simulink model "bh_explore_car_eom"  (R2017b)
settings: Solver=ode45  StartTime=0.0  StopTime=30  FixedStep=0.001  RelTol=1e-5
undefined symbols (not defined in the file or in its folder): sigbuilder_block, veh
libraries: simulink_extras x15, bh_cv_car_drc_library x1
settings Model: Creator=bhorton  LastModifiedBy=bhorton
settings SolverCC: ZeroCrossControl=EnableAll  ZeroCrossAlgorithm=Adaptive
settings DebuggingCC: SignalInfNanChecking=warning
settings ModelReferenceCC: ModelReferenceMinAlgLoopOccurrences=on

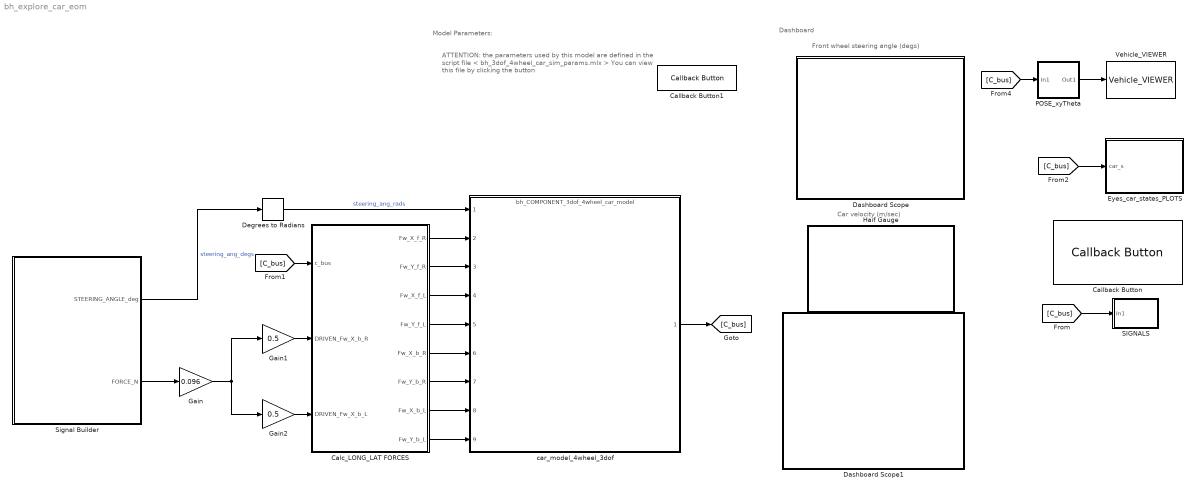
== system bh_explore_car_eom ==
  note: Car velocity (m/sec)
  note: ATTENTION:
      | the parameters used by this model are defined in the script file
      | < bh_3dof_4wheel_car_sim_params.mlx >
      |
      | You can view this file by clicking the button
  note: Model Parameters:
  note: Dashboard
  note: Front wheel steering angle (degs)
  Calc_LONG_LAT FORCES : Subsystem
  Callback Button : CallbackButton  WebBlockId=1673  PressFcn=""  ButtonText=OPEN State Plots  PressDelay=500  RepeatInterval=0
      settings: ClickFcn=|
      | open_system([bdroot,'/Eyes_car_states_PLOTS/car_states'])
      | open_system([bdroot,'/Eyes_car_states_PLOTS/Forces_BODY_frame'])
  Callback Button1 : CallbackButton  WebBlockId=1872  ButtonText=view parameter file  PressDelay=500  RepeatInterval=0
      settings: ClickFcn=edit bh_3dof_4wheel_car_sim_params.mlx
  Dashboard Scope : Subsystem  DialogController=hmiCreateDDGDialog  IsWebBlock=on  mask(MWDashboardBlock){webBlockId=37415055-6488-43ff-9aef-d1c13ce01a1d, webBlockType=sdiscope, ShowInitialText=on, HMISrcModelName=bh_explore_car_eom}
      mask prompts: webBlockId "WebBlock Id"; webBlockType "WebBlock Type"; HMISrcModelName "Source Model"
      mask help: SimulinkHMI:dialogs:HMIScopeDialogDesc
      mask Help: helpview([docroot '/mapfiles/simulink.map'], 'hmi_scope')
      mask Display:
      | if strcmp(get_param(bdroot(gcb),'BlockDiagramType'), 'library')
      |     image([(matlabroot) '/toolbox/simulink/hmi/icons/DashboardScope.png']);
      | end
  Dashboard Scope1 : Subsystem  DialogController=hmiCreateDDGDialog  IsWebBlock=on  mask(MWDashboardBlock){webBlockId=0f87227d-f9f9-4bc4-b6ae-007699aa5c2c, webBlockType=sdiscope, ShowInitialText=on, HMISrcModelName=bh_explore_car_eom}
      mask prompts: webBlockId "WebBlock Id"; webBlockType "WebBlock Type"; HMISrcModelName "Source Model"
      mask help: SimulinkHMI:dialogs:HMIScopeDialogDesc
      mask Help: helpview([docroot '/mapfiles/simulink.map'], 'hmi_scope')
      mask Display:
      | if strcmp(get_param(bdroot(gcb),'BlockDiagramType'), 'library')
      |     image([(matlabroot) '/toolbox/simulink/hmi/icons/DashboardScope.png']);
      | end
  Degrees to Radians : simulink_extras/Transformations/Degrees to Radians
  Eyes_car_states_PLOTS : Subsystem
  Gain : Gain  Gain=0.096
  Gain1 : Gain  Gain=0.5
  Gain2 : Gain  Gain=0.5
  Half Gauge : Subsystem  DialogController=hmiCreateDDGDialog  IsWebBlock=on  mask(MWDashboardBlock){webBlockId=0ce8c2a9-cad4-4196-9a6a-b4237871358c, webBlockType=semicirculargauge, ShowInLibBrowser=on, ShowInitialText=on, HMISrcModelName=bh_explore_car_eom}
      mask prompts: webBlockId "WebBlock Id"; webBlockType "WebBlock Type"; HMISrcModelName "Source Model"
      mask help: SimulinkHMI:dialogs:SemicircularGaugeDialogDesc
      mask Help: helpview([docroot '/mapfiles/simulink.map'], 'hmi_half_gauge')
      mask Display:
      | if strcmp(get_param(bdroot(gcb),'BlockDiagramType'), 'library')
      |     image([(matlabroot) '/toolbox/simulink/hmi/icons/SemicircularGauge.png']);
      | end
  POSE_xyTheta : Subsystem
  SIGNALS : Subsystem
  Signal Builder : Subsystem  Tag=STV Subsys  LoadFcn=sigbuilder_block('load');  StartFcn=sigbuilder_block('start');  StopFcn=sigbuilder_block('stop');  ClipboardFcn=sigbuilder_block('clipboard');  mask(Sigbuilder block){tuvar=[0:10]}
      mask help: Simulink:masks:SigbuilderBlock_MD
      mask init:
      | if ~strcmp(get_param(bdroot(gcbh),'SimulationStatus'),'stopped') tuvar = sigbuilder_block('maskInit'); end
      settings: CopyFcn=sigbuilder_block('copy');  DeleteFcn=sigbuilder_block('delete');  ModelCloseFcn=sigbuilder_block('modelClose');  PreSaveFcn=sigbuilder_block('preSave');  PauseFcn=sigbuilder_block('pause');  ContinueFcn=sigbuilder_block('continue');  NameChangeFcn=sigbuilder_block('namechange');  OpenFcn=sigbuilder_block('open',[437.6 199.2 550.4 400 ]);  CloseFcn=sigbuilder_block('close');
      mask Display: plot(0, 0, 100, 100,[2, 2, 32, 32, 2], [68, 8, 8, 68, 68],[32, 2], [38, 38], [32, 19, 2],[53, 60, 44], [32, 17, 17, 2],[16, 16, 31, 31]);txt = getActiveGroup(gcbh);text(2, 100, txt,'verticalAlignment', 'top');
  Vehicle_VIEWER : bh_cv_car_drc_library/CAR_things/Vehicle_VIEWER  wp_mat=[-1, -1; 2,2]  veh_ID_num=1  veh_init_xytheta=[0,0,0]  Ts=0.1
  car_model_4wheel_3dof : ModelReference  ModelNameDialog=bh_COMPONENT_3dof_4wheel_car_model.slx  SimulationMode=Normal  ModelReferenceVersion=1.187
  wires:
  [C_bus] -> Eyes_car_states_PLOTS/1(car_s)
  car_model_4wheel_3dof/1 -> [C_bus]
  [C_bus] -> POSE_xyTheta/1(In1)
  POSE_xyTheta/1(Out1) -> Vehicle_VIEWER/1
  [C_bus] -> SIGNALS/1(In1)
  Calc_LONG_LAT FORCES/8(Fw_Y_b_L) -> car_model_4wheel_3dof/9
  Calc_LONG_LAT FORCES/1(Fw_X_f_R) -> car_model_4wheel_3dof/2
  Calc_LONG_LAT FORCES/2(Fw_Y_f_R) -> car_model_4wheel_3dof/3
  Calc_LONG_LAT FORCES/3(Fw_X_f_L) -> car_model_4wheel_3dof/4
  Calc_LONG_LAT FORCES/4(Fw_Y_f_L) -> car_model_4wheel_3dof/5
  Calc_LONG_LAT FORCES/5(Fw_X_b_R) -> car_model_4wheel_3dof/6
  Calc_LONG_LAT FORCES/6(Fw_Y_b_R) -> car_model_4wheel_3dof/7
  Calc_LONG_LAT FORCES/7(Fw_X_b_L) -> car_model_4wheel_3dof/8
  [C_bus] -> Calc_LONG_LAT FORCES/1(c_bus)
  Degrees to Radians/1 -> car_model_4wheel_3dof/1  "steering_ang_rads"
  Gain/1 -> Gain1/1, Gain2/1
  Gain1/1 -> Calc_LONG_LAT FORCES/2(DRIVEN_Fw_X_b_R)
  Gain2/1 -> Calc_LONG_LAT FORCES/3(DRIVEN_Fw_X_b_L)
  Signal Builder/1(STEERING_ANGLE_deg) -> Degrees to Radians/1  "steering_ang_degs"
  Signal Builder/2(FORCE_N) -> Gain/1

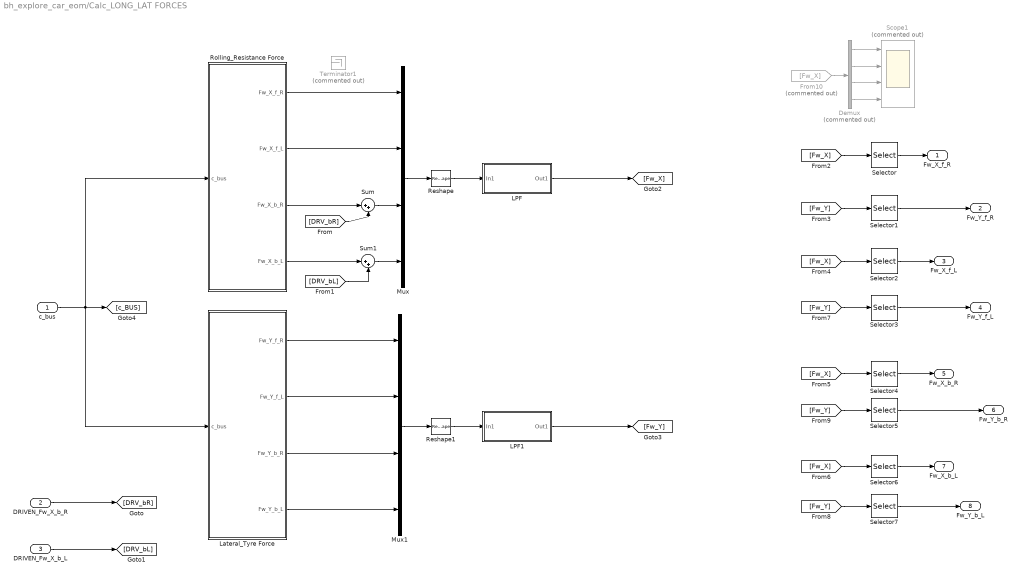
== system bh_explore_car_eom/Calc_LONG_LAT FORCES ==
  c_bus : Inport
  DRIVEN_Fw_X_b_R : Inport  Port=2
  DRIVEN_Fw_X_b_L : Inport  Port=3
  Demux : Demux  Commented=on
  From10 : From  Commented=on  GotoTag=Fw_X
  LPF : Subsystem
  LPF1 : Subsystem
  Lateral_Tyre Force : Subsystem
  Mux : Mux
  Mux1 : Mux
  Reshape : Reshape  OutputDimensionality=Column vector (2-D)
  Reshape1 : Reshape  OutputDimensionality=Column vector (2-D)
  Rolling_Resistance Force : Subsystem
  Scope1 : Scope  Commented=on  NumInputPorts=4
  Selector : Selector  InputPortWidth=4  IndexOptions=Index vector (dialog)  Indices=1  OutputSizes=1
  Selector1 : Selector  InputPortWidth=4  IndexOptions=Index vector (dialog)  Indices=1  OutputSizes=1
  Selector2 : Selector  InputPortWidth=4  IndexOptions=Index vector (dialog)  Indices=2  OutputSizes=1
  Selector3 : Selector  InputPortWidth=4  IndexOptions=Index vector (dialog)  Indices=2  OutputSizes=1
  Selector4 : Selector  InputPortWidth=4  IndexOptions=Index vector (dialog)  Indices=3  OutputSizes=1
  Selector5 : Selector  InputPortWidth=4  IndexOptions=Index vector (dialog)  Indices=3  OutputSizes=1
  Selector6 : Selector  InputPortWidth=4  IndexOptions=Index vector (dialog)  Indices=4  OutputSizes=1
  Selector7 : Selector  InputPortWidth=4  IndexOptions=Index vector (dialog)  Indices=4  OutputSizes=1
  Sum : Sum  Inputs=|++
  Sum1 : Sum  Inputs=|++
  Terminator1 : Terminator  Commented=on
  Fw_X_f_R : Outport
  Fw_Y_f_R : Outport  Port=2
  Fw_X_f_L : Outport  Port=3
  Fw_Y_f_L : Outport  Port=4
  Fw_X_b_R : Outport  Port=5
  Fw_Y_b_R : Outport  Port=6
  Fw_X_b_L : Outport  Port=7
  Fw_Y_b_L : Outport  Port=8
  wires:
  Selector/1 -> Fw_X_f_R/1
  Selector5/1 -> Fw_Y_b_R/1
  Selector7/1 -> Fw_Y_b_L/1
  Selector1/1 -> Fw_Y_f_R/1
  c_bus/1 -> [c_BUS], Rolling_Resistance Force/1(c_bus), Lateral_Tyre Force/1(c_bus)
  DRIVEN_Fw_X_b_R/1 -> [DRV_bR]
  DRIVEN_Fw_X_b_L/1 -> [DRV_bL]
  Rolling_Resistance Force/2(Fw_X_f_L) -> Mux/2
  Rolling_Resistance Force/1(Fw_X_f_R) -> Mux/1
  Lateral_Tyre Force/1(Fw_Y_f_R) -> Mux1/1
  Lateral_Tyre Force/2(Fw_Y_f_L) -> Mux1/2
  Lateral_Tyre Force/3(Fw_Y_b_R) -> Mux1/3
  Lateral_Tyre Force/4(Fw_Y_b_L) -> Mux1/4
  Mux1/1 -> Reshape1/1
  Mux/1 -> Reshape/1
  [Fw_Y] -> Selector1/1
  [Fw_X] -> Selector/1
  Selector6/1 -> Fw_X_b_L/1
  Selector4/1 -> Fw_X_b_R/1
  Selector3/1 -> Fw_Y_f_L/1
  Selector2/1 -> Fw_X_f_L/1
  [Fw_Y] -> Selector7/1
  [Fw_X] -> Selector6/1
  [Fw_Y] -> Selector5/1
  [Fw_X] -> Selector4/1
  [Fw_Y] -> Selector3/1
  [Fw_X] -> Selector2/1
  Reshape/1 -> LPF/1(In1)
  LPF/1(Out1) -> [Fw_X]
  LPF1/1(Out1) -> [Fw_Y]
  Demux/1 -> Scope1/1
  Demux/2 -> Scope1/2
  Demux/3 -> Scope1/3
  Demux/4 -> Scope1/4
  From10/1 -> Demux/1
  Rolling_Resistance Force/3(Fw_X_b_R) -> Sum/1
  [DRV_bR] -> Sum/2
  Sum1/1 -> Mux/4
  Rolling_Resistance Force/4(Fw_X_b_L) -> Sum1/1
  [DRV_bL] -> Sum1/2
  Sum/1 -> Mux/3
  Reshape1/1 -> LPF1/1(In1)

== system bh_explore_car_eom/Dashboard Scope ==

== system bh_explore_car_eom/Dashboard Scope1 ==

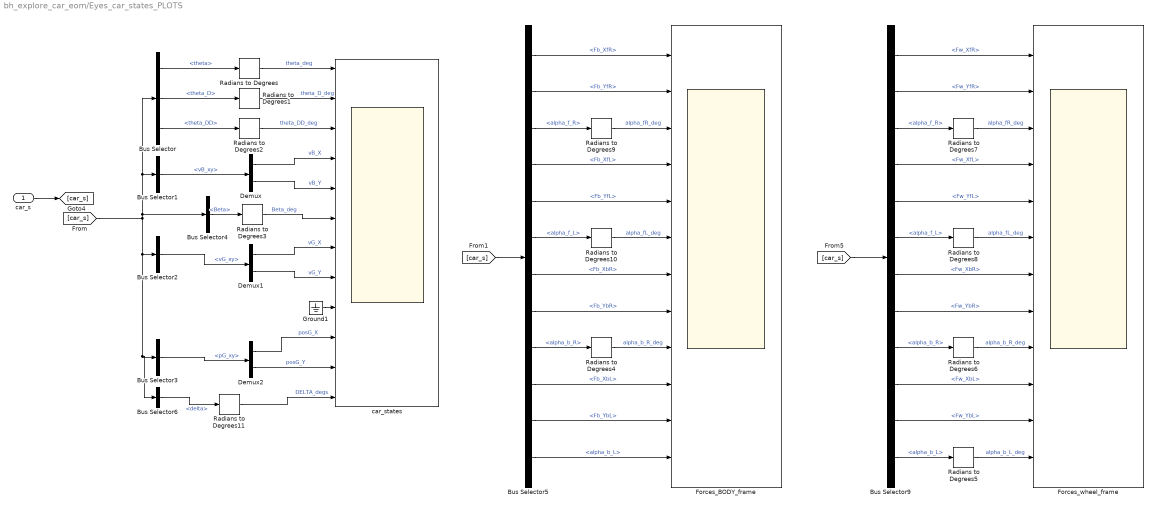
== system bh_explore_car_eom/Eyes_car_states_PLOTS ==
  car_s : Inport
  Bus Selector : BusSelector  OutputSignals=states_B.theta,states_B.theta_D,states_B.theta_DD
  Bus Selector1 : BusSelector  OutputSignals=states_B.vB_xy
  Bus Selector2 : BusSelector  OutputSignals=states_G.vG_xy
  Bus Selector3 : BusSelector  OutputSignals=states_G.pG_xy
  Bus Selector4 : BusSelector  OutputSignals=states_B.Beta
  Bus Selector5 : BusSelector  OutputSignals=Force_BODY_frame.Fb_XfR,Force_BODY_frame.Fb_YfR,alpha.alpha_f_R,Force_BODY_frame.Fb_XfL,Force_BODY_frame.Fb_YfL,alpha.alpha_f_L,Force_BODY_frame.Fb_XbR,Force_BODY_frame.Fb_YbR,alpha.alpha_b_R,Force_BODY_frame.Fb_XbL,Force_BODY_frame.Fb_YbL,alpha.alpha_b_L
  Bus Selector6 : BusSelector  OutputSignals=wheel.delta
  Bus Selector9 : BusSelector  OutputSignals=Force_wheel_frame.Fw_XfR,Force_wheel_frame.Fw_YfR,alpha.alpha_f_R,Force_wheel_frame.Fw_XfL,Force_wheel_frame.Fw_YfL,alpha.alpha_f_L,Force_wheel_frame.Fw_XbR,Force_wheel_frame.Fw_YbR,alpha.alpha_b_R,Force_wheel_frame.Fw_XbL,Force_wheel_frame.Fw_YbL,alpha.alpha_b_L
  Demux : Demux  Outputs=2
  Demux1 : Demux  Outputs=2
  Demux2 : Demux  Outputs=2
  Forces_BODY_frame : Scope  NumInputPorts=12
  Forces_wheel_frame : Scope  NumInputPorts=12
  Ground1 : Ground
  Radians to Degrees{,1..11} (12 alike) : simulink_extras/Transformations/Radians to Degrees
  car_states : Scope  NumInputPorts=12
  wires:
  car_s/1 -> [car_s]
  [car_s] -> Bus Selector4/1, Bus Selector/1, Bus Selector1/1, Bus Selector6/1, Bus Selector3/1, Bus Selector2/1
  Bus Selector/1 -> Radians to Degrees/1  "<theta>"
  Bus Selector/2 -> Radians to Degrees1/1  "<theta_D>"
  Bus Selector/3 -> Radians to Degrees2/1  "<theta_DD>"
  Radians to Degrees/1 -> car_states/1  "theta_deg"
  Radians to Degrees1/1 -> car_states/2  "theta_D_deg"
  Radians to Degrees2/1 -> car_states/3  "theta_DD_deg"
  Bus Selector1/1 -> Demux/1  "<vB_xy>"
  Demux/1 -> car_states/4  "vB_X"
  Demux/2 -> car_states/5  "vB_Y"
  Radians to Degrees3/1 -> car_states/6  "Beta_deg"
  Bus Selector2/1 -> Demux1/1  "<vG_xy>"
  Demux1/1 -> car_states/7  "vG_X"
  Demux1/2 -> car_states/8  "vG_Y"
  Ground1/1 -> car_states/9
  Demux2/1 -> car_states/10  "posG_X"
  Demux2/2 -> car_states/11  "posG_Y"
  Bus Selector3/1 -> Demux2/1  "<pG_xy>"
  Radians to Degrees11/1 -> car_states/12  "DELTA_degs"
  Bus Selector4/1 -> Radians to Degrees3/1  "<Beta>"
  [car_s] -> Bus Selector9/1
  Bus Selector9/1 -> Forces_wheel_frame/1  "<Fw_XfR>"
  Bus Selector9/2 -> Forces_wheel_frame/2  "<Fw_YfR>"
  Bus Selector9/3 -> Radians to Degrees7/1  "<alpha_f_R>"
  Bus Selector9/4 -> Forces_wheel_frame/4  "<Fw_XfL>"
  Bus Selector9/5 -> Forces_wheel_frame/5  "<Fw_YfL>"
  Bus Selector9/6 -> Radians to Degrees8/1  "<alpha_f_L>"
  Bus Selector9/7 -> Forces_wheel_frame/7  "<Fw_XbR>"
  Bus Selector9/8 -> Forces_wheel_frame/8  "<Fw_YbR>"
  Bus Selector9/9 -> Radians to Degrees6/1  "<alpha_b_R>"
  Bus Selector9/10 -> Forces_wheel_frame/10  "<Fw_XbL>"
  Bus Selector9/11 -> Forces_wheel_frame/11  "<Fw_YbL>"
  Bus Selector9/12 -> Radians to Degrees5/1  "<alpha_b_L>"
  Radians to Degrees7/1 -> Forces_wheel_frame/3  "alpha_fR_deg"
  Radians to Degrees8/1 -> Forces_wheel_frame/6  "alpha_fL_deg"
  Radians to Degrees6/1 -> Forces_wheel_frame/9  "alpha_b_R_deg"
  Radians to Degrees5/1 -> Forces_wheel_frame/12  "alpha_b_L_deg"
  Radians to Degrees10/1 -> Forces_BODY_frame/6  "alpha_fL_deg"
  Radians to Degrees4/1 -> Forces_BODY_frame/9  "alpha_b_R_deg"
  Radians to Degrees9/1 -> Forces_BODY_frame/3  "alpha_fR_deg"
  Bus Selector5/9 -> Radians to Degrees4/1  "<alpha_b_R>"
  Bus Selector5/7 -> Forces_BODY_frame/7  "<Fb_XbR>"
  Bus Selector5/10 -> Forces_BODY_frame/10  "<Fb_XbL>"
  Bus Selector5/11 -> Forces_BODY_frame/11  "<Fb_YbL>"
  Bus Selector5/6 -> Radians to Degrees10/1  "<alpha_f_L>"
  Bus Selector5/5 -> Forces_BODY_frame/5  "<Fb_YfL>"
  Bus Selector5/4 -> Forces_BODY_frame/4  "<Fb_XfL>"
  Bus Selector5/8 -> Forces_BODY_frame/8  "<Fb_YbR>"
  Bus Selector5/2 -> Forces_BODY_frame/2  "<Fb_YfR>"
  [car_s] -> Bus Selector5/1
  Bus Selector5/3 -> Radians to Degrees9/1  "<alpha_f_R>"
  Bus Selector5/1 -> Forces_BODY_frame/1  "<Fb_XfR>"
  Bus Selector5/12 -> Forces_BODY_frame/12  "<alpha_b_L>"
  Bus Selector6/1 -> Radians to Degrees11/1  "<delta>"

== system bh_explore_car_eom/Half Gauge ==

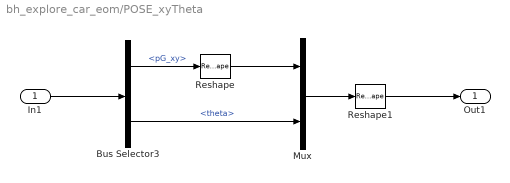
== system bh_explore_car_eom/POSE_xyTheta ==
  In1 : Inport
  Bus Selector3 : BusSelector  OutputSignals=states_G.pG_xy,states_B.theta
  Mux : Mux  Inputs=2
  Reshape : Reshape  OutputDimensionality=Column vector (2-D)
  Reshape1 : Reshape  OutputDimensionality=Column vector (2-D)
  Out1 : Outport
  wires:
  In1/1 -> Bus Selector3/1
  Bus Selector3/1 -> Reshape/1  "<pG_xy>"
  Reshape/1 -> Mux/1
  Bus Selector3/2 -> Mux/2  "<theta>"
  Mux/1 -> Reshape1/1
  Reshape1/1 -> Out1/1

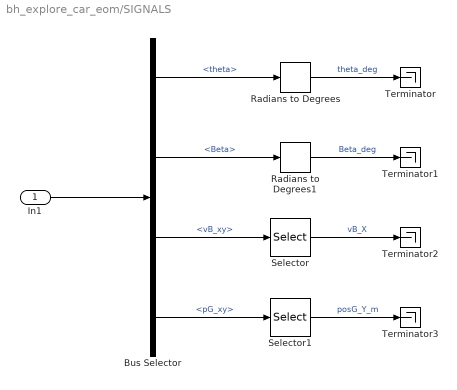
== system bh_explore_car_eom/SIGNALS ==
  In1 : Inport
  Bus Selector : BusSelector  OutputSignals=states_B.theta,states_B.Beta,states_B.vB_xy,states_G.pG_xy
  Radians to Degrees : simulink_extras/Transformations/Radians to Degrees
  Radians to Degrees1 : simulink_extras/Transformations/Radians to Degrees
  Selector : Selector  InputPortWidth=2  IndexOptions=Index vector (dialog)  Indices=1  OutputSizes=1
  Selector1 : Selector  InputPortWidth=2  IndexOptions=Index vector (dialog)  Indices=2  OutputSizes=1
  Terminator{,1..3} (4 alike) : Terminator
  wires:
  In1/1 -> Bus Selector/1
  Bus Selector/1 -> Radians to Degrees/1  "<theta>"
  Bus Selector/2 -> Radians to Degrees1/1  "<Beta>"
  Bus Selector/3 -> Selector/1  "<vB_xy>"
  Selector/1 -> Terminator2/1  "vB_X"
  Bus Selector/4 -> Selector1/1  "<pG_xy>"
  Selector1/1 -> Terminator3/1  "posG_Y_m"
  Radians to Degrees/1 -> Terminator/1  "theta_deg"
  Radians to Degrees1/1 -> Terminator1/1  "Beta_deg"

== system bh_explore_car_eom/Signal Builder ==
  Demux : Demux  Tag=STV Demux  Outputs=2
  FromWs : FromWorkspace  Tag=STV FromWs  VariableName=tuvar  SampleTime=0
      SigBuilderData=|
      | common.afterFinalStr = 'Extrapolate'
      | common.sampleTime = 0
      | dataSet(1).timeRange = [0 10]
      | dataSet(1).name = 'Drive_STRAIGHT'
      | dataSet(2).timeRange = [0 15]
      | dataSet(2).name = 'Drive_LOCK'
      | dataSet(3).timeRange = [0 45]
      | dataSet(3).name = 'Drive_TURN'
      | sbobj.Groups(1).Name = 'Drive_STRAIGHT'
      | sbobj.Groups(1).Signals(1).Name = 'STEERING_ANGLE_deg'
      | sbobj.Groups(1).Signals(1).XData = [0 3 10]
      | sbobj.Groups(1).Signals(1).YData = [0 0 0]
      | sbobj.Groups(1).Signals(2).Name = 'FORCE_N'
      | sbobj.Groups(1).Signals(2).XData = [0 3 3 5.98 5.98 10]
      | sbobj.Groups(1).Signals(2).YData = [0 0 3 3 1 1]
      | sbobj.Groups(2).Name = 'Drive_LOCK'
      | sbobj.Groups(2).Signals(1).Name = 'STEERING_ANGLE_deg'
      | sbobj.Groups(2).Signals(1).XData = [0 3 10 10 15]
      | sbobj.Groups(2).Signals(1).YData = [0 0 0 25 25]
      | sbobj.Groups(2).Signals(2).Name = 'FORCE_N'
      | sbobj.Groups(2).Signals(2).XData = [0 3 3 5.98 5.98 15]
      | sbobj.Groups(2).Signals(2).YData = [0 0 3 3 1 1]
      | sbobj.Groups(2).TimeRange = [0 15]
      | sbobj.Groups(3).Name = 'Drive_TURN'
      | sbobj.Groups(3).Signals(1).Name = 'STEERING_ANGLE_deg'
      | sbobj.Groups(3).Signals(1).XData = [0 3 10 10 13 13 45]
      | sbobj.Groups(3).Signals(1).YData = [0 0 0 25 25 0 0]
      | sbobj.Groups(3).Signals(2).Name = 'FORCE_N'
      | sbobj.Groups(3).Signals(2).XData = [0 3 3 5.98 5.98 45]
      | sbobj.Groups(3).Signals(2).YData = [0 0 3 3 1 1]
      | sbobj.Groups(3).TimeRange = [0 45]
  STEERING_ANGLE_deg : Outport  Tag=STV Outport
  FORCE_N : Outport  Tag=STV Outport  Port=2
  wires:
  FromWs/1 -> Demux/1
  Demux/1 -> STEERING_ANGLE_deg/1
  Demux/2 -> FORCE_N/1

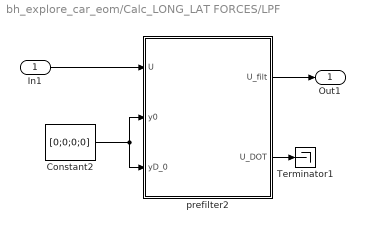
== system bh_explore_car_eom/Calc_LONG_LAT FORCES/LPF ==
  In1 : Inport
  Constant2 : Constant  Value=[0;0;0;0]  VectorParams1D=off
  Terminator1 : Terminator
  prefilter2 : Subsystem  mask(Derivative Estimation){wn=2*pi*100, p=1}
      mask prompts: wn "Natural frequency, wn (rad/sec)"; p "Damping ratio, p"
      mask help:
      | A simple derivative estimator using a 2nd order representation between input and output.
      |
      | The integrators use a discrete FORWARd Euler rule, and a sample time needs to be specified.
      mask init:
      | str1 = sprintf('wn = %.2f', wn);
      | str2 = sprintf('p  = %.2f', p);
      | %str3 = sprintf('dt = %.2f', dt);
      | %str = char(str1,str2,str3);
      | %str3 = sprintf('dt = %.2f', dt);
      | str = char(str1,str2);
      mask Display: disp(str)
  Out1 : Outport
  wires:
  prefilter2/2(U_DOT) -> Terminator1/1
  Constant2/1 -> prefilter2/2(y0), prefilter2/3(yD_0)
  prefilter2/1(U_filt) -> Out1/1
  In1/1 -> prefilter2/1(U)

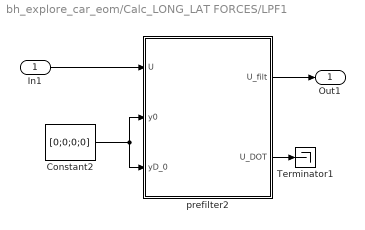
== system bh_explore_car_eom/Calc_LONG_LAT FORCES/LPF1 ==
  In1 : Inport
  Constant2 : Constant  Value=[0;0;0;0]  VectorParams1D=off
  Terminator1 : Terminator
  prefilter2 : Subsystem  mask(Derivative Estimation){wn=2*pi*100, p=1}
      mask prompts: wn "Natural frequency, wn (rad/sec)"; p "Damping ratio, p"
      mask help:
      | A simple derivative estimator using a 2nd order representation between input and output.
      |
      | The integrators use a discrete FORWARd Euler rule, and a sample time needs to be specified.
      mask init:
      | str1 = sprintf('wn = %.2f', wn);
      | str2 = sprintf('p  = %.2f', p);
      | %str3 = sprintf('dt = %.2f', dt);
      | %str = char(str1,str2,str3);
      | %str3 = sprintf('dt = %.2f', dt);
      | str = char(str1,str2);
      mask Display: disp(str)
  Out1 : Outport
  wires:
  prefilter2/2(U_DOT) -> Terminator1/1
  Constant2/1 -> prefilter2/2(y0), prefilter2/3(yD_0)
  prefilter2/1(U_filt) -> Out1/1
  In1/1 -> prefilter2/1(U)

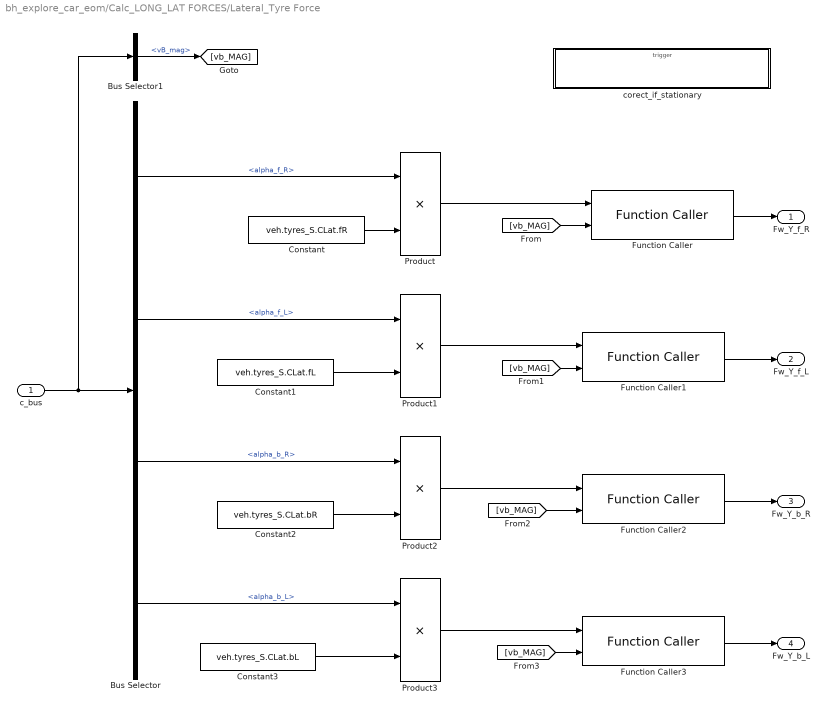
== system bh_explore_car_eom/Calc_LONG_LAT FORCES/Lateral_Tyre Force ==
  c_bus : Inport
  Bus Selector : BusSelector  OutputSignals=alpha.alpha_f_R,alpha.alpha_f_L,alpha.alpha_b_R,alpha.alpha_b_L
  Bus Selector1 : BusSelector  OutputSignals=states_B.vB_mag
  Constant : Constant  Value=veh.tyres_S.CLat.fR
  Constant1 : Constant  Value=veh.tyres_S.CLat.fL
  Constant2 : Constant  Value=veh.tyres_S.CLat.bR
  Constant3 : Constant  Value=veh.tyres_S.CLat.bL
  Function Caller{,1..3} (4 alike) : FunctionCaller  FunctionPrototype=y = correct_if_stationary(Fw_Y,vb_MAG)  InputArgumentSpecifications=double(1), double(1)  OutputArgumentSpecifications=double(1)
  Product{,1..3} (4 alike) : Product
  corect_if_stationary : Subsystem  TreatAsAtomicUnit=on
  Fw_Y_f_R : Outport
  Fw_Y_f_L : Outport  Port=2
  Fw_Y_b_R : Outport  Port=3
  Fw_Y_b_L : Outport  Port=4
  wires:
  c_bus/1 -> Bus Selector1/1, Bus Selector/1
  Bus Selector/1 -> Product/1  "<alpha_f_R>"
  Constant/1 -> Product/2
  Bus Selector/2 -> Product1/1  "<alpha_f_L>"
  Constant1/1 -> Product1/2
  Bus Selector/3 -> Product2/1  "<alpha_b_R>"
  Constant2/1 -> Product2/2
  Bus Selector/4 -> Product3/1  "<alpha_b_L>"
  Constant3/1 -> Product3/2
  Bus Selector1/1 -> [vb_MAG]  "<vB_mag>"
  Product/1 -> Function Caller/1
  Function Caller/1 -> Fw_Y_f_R/1
  Function Caller1/1 -> Fw_Y_f_L/1
  Function Caller2/1 -> Fw_Y_b_R/1
  Function Caller3/1 -> Fw_Y_b_L/1
  [vb_MAG] -> Function Caller/2
  Product1/1 -> Function Caller1/1
  Product2/1 -> Function Caller2/1
  Product3/1 -> Function Caller3/1
  [vb_MAG] -> Function Caller1/2
  [vb_MAG] -> Function Caller2/2
  [vb_MAG] -> Function Caller3/2

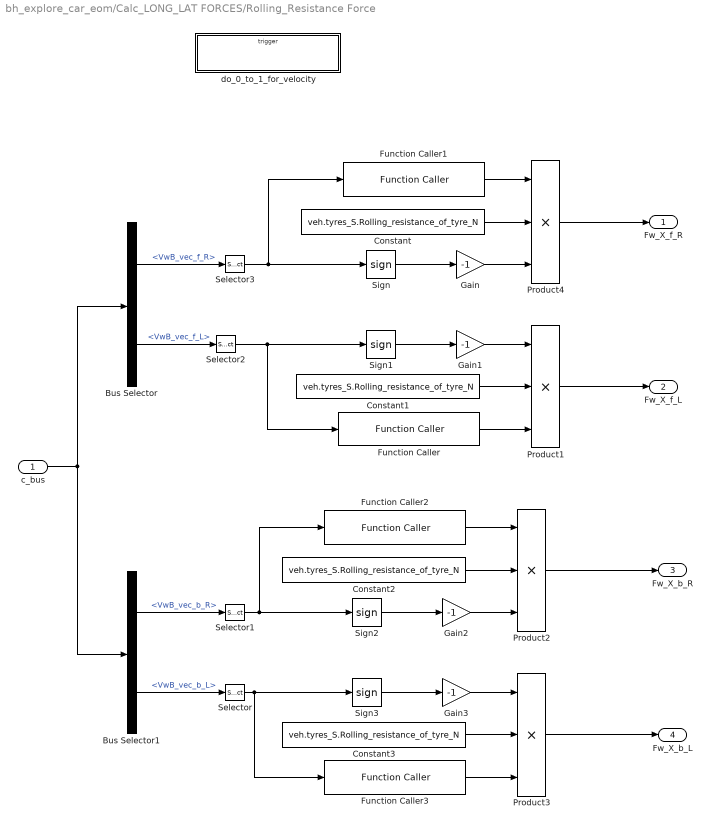
== system bh_explore_car_eom/Calc_LONG_LAT FORCES/Rolling_Resistance Force ==
  c_bus : Inport
  Bus Selector : BusSelector  OutputSignals=wheel.VwB_vec_f_R,wheel.VwB_vec_f_L
  Bus Selector1 : BusSelector  OutputSignals=wheel.VwB_vec_b_R,wheel.VwB_vec_b_L
  Constant{,1..3} (4 alike) : Constant  Value=veh.tyres_S.Rolling_resistance_of_tyre_N
  Function Caller{,1..3} (4 alike) : FunctionCaller  FunctionPrototype=y = zero_to_1_from_VEL(u)  InputArgumentSpecifications=double(1)  OutputArgumentSpecifications=double(1)
  Gain{,1..3} (4 alike) : Gain  Gain=-1
  Product{1..4} (4 alike) : Product  Inputs=3
  Selector{,1..3} (4 alike) : Selector  InputPortWidth=2  IndexOptions=Index vector (dialog)  Indices=1  OutputSizes=1
  Sign{,1..3} (4 alike) : Signum
  do_0_to_1_for_velocity : Subsystem  TreatAsAtomicUnit=on
  Fw_X_f_R : Outport
  Fw_X_f_L : Outport  Port=2
  Fw_X_b_R : Outport  Port=3
  Fw_X_b_L : Outport  Port=4
  wires:
  c_bus/1 -> Bus Selector1/1, Bus Selector/1
  Bus Selector/1 -> Selector3/1  "<VwB_vec_f_R>"
  Bus Selector/2 -> Selector2/1  "<VwB_vec_f_L>"
  Sign/1 -> Gain/1
  Sign1/1 -> Gain1/1
  Gain/1 -> Product4/3
  Gain1/1 -> Product1/1
  Constant/1 -> Product4/2
  Constant1/1 -> Product1/2
  Product1/1 -> Fw_X_f_L/1
  Product4/1 -> Fw_X_f_R/1
  Gain2/1 -> Product2/3
  Sign3/1 -> Gain3/1
  Gain3/1 -> Product3/1
  Bus Selector1/1 -> Selector1/1  "<VwB_vec_b_R>"
  Constant2/1 -> Product2/2
  Sign2/1 -> Gain2/1
  Product3/1 -> Fw_X_b_L/1
  Product2/1 -> Fw_X_b_R/1
  Constant3/1 -> Product3/2
  Bus Selector1/2 -> Selector/1  "<VwB_vec_b_L>"
  Function Caller/1 -> Product1/3
  Function Caller1/1 -> Product4/1
  Function Caller2/1 -> Product2/1
  Function Caller3/1 -> Product3/3
  Selector3/1 -> Function Caller1/1, Sign/1
  Selector2/1 -> Function Caller/1, Sign1/1
  Selector1/1 -> Function Caller2/1, Sign2/1
  Selector/1 -> Function Caller3/1, Sign3/1

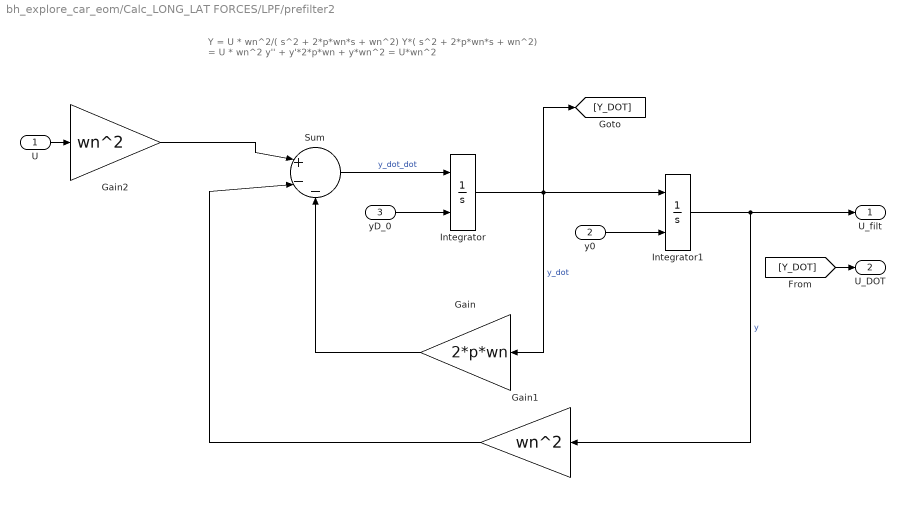
== system bh_explore_car_eom/Calc_LONG_LAT FORCES/LPF/prefilter2 ==
  note: Y = U *     wn^2/( s^2 + 2*p*wn*s + wn^2)
      | Y*( s^2 + 2*p*wn*s + wn^2) = U * wn^2
      |
      | y'' + y'*2*p*wn + y*wn^2 = U*wn^2
  U : Inport
  y0 : Inport  Port=2
  yD_0 : Inport  Port=3
  Gain : Gain  Gain=2*p*wn
  Gain1 : Gain  Gain=wn^2
  Gain2 : Gain  Gain=wn^2
  Integrator : Integrator  InitialConditionSource=external
  Integrator1 : Integrator  InitialConditionSource=external
  Sum : Sum  Inputs=|+--
  U_filt : Outport
  U_DOT : Outport  Port=2
  wires:
  Integrator/1 -> [Y_DOT], Gain/1, Integrator1/1  "y_dot"
  Sum/1 -> Integrator/1  "y_dot_dot"
  Integrator1/1 -> Gain1/1, U_filt/1  "y"
  U/1 -> Gain2/1
  Gain2/1 -> Sum/1
  Gain/1 -> Sum/3
  Gain1/1 -> Sum/2
  [Y_DOT] -> U_DOT/1
  yD_0/1 -> Integrator/2
  y0/1 -> Integrator1/2

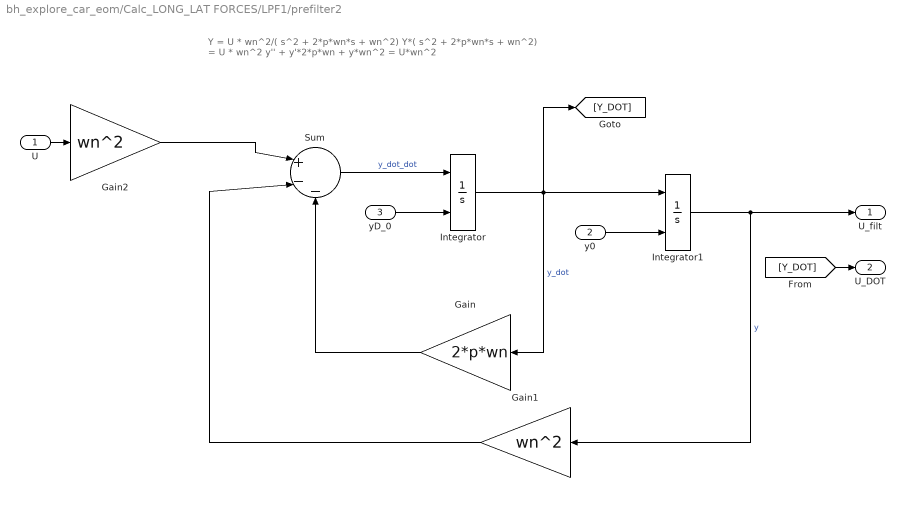
== system bh_explore_car_eom/Calc_LONG_LAT FORCES/LPF1/prefilter2 ==
  note: Y = U *     wn^2/( s^2 + 2*p*wn*s + wn^2)
      | Y*( s^2 + 2*p*wn*s + wn^2) = U * wn^2
      |
      | y'' + y'*2*p*wn + y*wn^2 = U*wn^2
  U : Inport
  y0 : Inport  Port=2
  yD_0 : Inport  Port=3
  Gain : Gain  Gain=2*p*wn
  Gain1 : Gain  Gain=wn^2
  Gain2 : Gain  Gain=wn^2
  Integrator : Integrator  InitialConditionSource=external
  Integrator1 : Integrator  InitialConditionSource=external
  Sum : Sum  Inputs=|+--
  U_filt : Outport
  U_DOT : Outport  Port=2
  wires:
  Integrator/1 -> [Y_DOT], Gain/1, Integrator1/1  "y_dot"
  Sum/1 -> Integrator/1  "y_dot_dot"
  Integrator1/1 -> Gain1/1, U_filt/1  "y"
  U/1 -> Gain2/1
  Gain2/1 -> Sum/1
  Gain/1 -> Sum/3
  Gain1/1 -> Sum/2
  [Y_DOT] -> U_DOT/1
  yD_0/1 -> Integrator/2
  y0/1 -> Integrator1/2

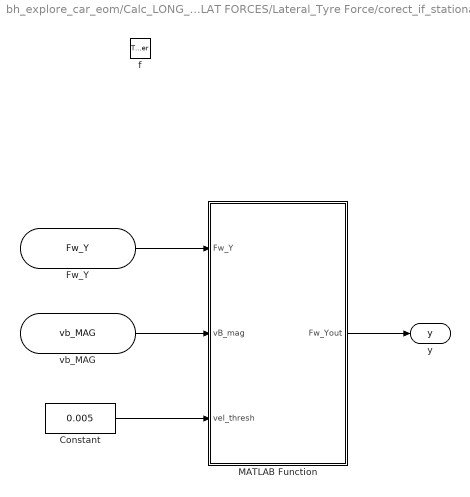
== system bh_explore_car_eom/Calc_LONG_LAT FORCES/Lateral_Tyre Force/corect_if_stationary ==
  f : TriggerPort  TriggerType=function-call  IsSimulinkFunction=on  FunctionName=correct_if_stationary  FunctionVisibility=scoped  VariantControl=(inherit)
  Constant : Constant  Value=0.005
  MATLAB Function : MATLAB Function  TreatAsAtomicUnit=on
  Fw_Y : ArgIn  DisableCoverage=on  ArgumentName=Fw_Y
  vb_MAG : ArgIn  DisableCoverage=on  Port=2  ArgumentName=vb_MAG
  y : ArgOut  DisableCoverage=on  ArgumentName=y
  wires:
  Fw_Y/1 -> MATLAB Function/1(Fw_Y)
  Constant/1 -> MATLAB Function/3(vel_thresh)
  vb_MAG/1 -> MATLAB Function/2(vB_mag)
  MATLAB Function/1(Fw_Yout) -> y/1

== system bh_explore_car_eom/Calc_LONG_LAT FORCES/Rolling_Resistance Force/do_0_to_1_for_velocity ==
  zero_to_1_from_VEL : TriggerPort  TriggerType=function-call  IsSimulinkFunction=on  FunctionName=zero_to_1_from_VEL  FunctionVisibility=scoped  VariantControl=(inherit)
  1-D Lookup Table : Lookup_n-D  NumberOfTableDimensions=1  BreakpointsForDimension1=[0, 0.005, 0.01]  Table=[0,1,1]  ExtrapMethod=Clip  InternalRulePriority=Speed  RndMeth=Simplest  InputSameDT=on
  Abs : Abs
  u : ArgIn  DisableCoverage=on  ArgumentName=u
  y : ArgOut  DisableCoverage=on  ArgumentName=y
  wires:
  Abs/1 -> 1-D Lookup Table/1
  1-D Lookup Table/1 -> y/1
  u/1 -> Abs/1

== matlab function bh_explore_car_eom/Calc_LONG_LAT FORCES/Lateral_Tyre Force/corect_if_stationary/MATLAB Function ==
  data: Fw_Y input; vB_mag input; vel_thresh input; Fw_Yout output
function Fw_Yout = fcn(Fw_Y, vB_mag, vel_thresh)

if(vB_mag <= vel_thresh)

     Fw_Yout =  0;
else
     Fw_Yout =  Fw_Y; 
end
